simulink model "modelo2"  (R2016a)
settings: Solver=VariableStepAuto  StartTime=0.0  StopTime=2000  RelTol=1e-3
libraries: simulink x2
settings Model: Creator=Brunno  LastModifiedBy=Brunno

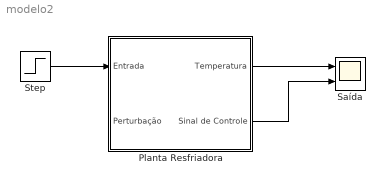
== system modelo2 ==
  Planta Resfriadora : Subsystem
  Saída : Scope  NumInputPorts=2
  Step : Step  Time=10  SampleTime=0
  wires:
  Step/1 -> Planta Resfriadora/1(Entrada)
  Planta Resfriadora/1(Temperatura) -> Saída/1
  Planta Resfriadora/2(Sinal de Controle) -> Saída/2

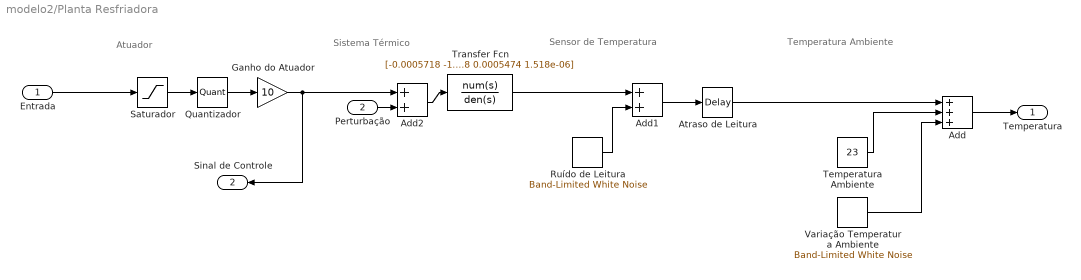
== system modelo2/Planta Resfriadora ==
  note: Temperatura Ambiente
  note: Sistema Térmico
  note: Atuador
  note: Sensor de Temperatura
  Entrada : Inport
  Perturbação : Inport  Port=2
  Add : Sum  Inputs=+++
  Add1 : Sum
  Add2 : Sum
  Atraso de Leitura : TransportDelay
  Ganho do Atuador : Gain  Gain=10
  Quantizador : Quantizer  QuantizationInterval=1/255
  Ruído de Leitura : simulink/Sources/Band-Limited White Noise  Cov=[0.001]  Ts=20  seed=[23341]
  Saturador : Saturate  UpperLimit=1  LowerLimit=0
  Temperatura Ambiente : Constant  Value=23
  Transfer Fcn : TransferFcn  Numerator=[-0.0005718 -1.226e-06]  Denominator=[1 0.04098 0.0005474 1.518e-06]
  Variação Temperatura Ambiente : simulink/Sources/Band-Limited White Noise  Cov=[1]  Ts=1000  seed=[23341]
  Temperatura : Outport
  Sinal de Controle : Outport  Port=2
  wires:
  Temperatura Ambiente/1 -> Add/2
  Entrada/1 -> Saturador/1
  Saturador/1 -> Quantizador/1
  Quantizador/1 -> Ganho do Atuador/1
  Variação Temperatura Ambiente/1 -> Add/3
  Atraso de Leitura/1 -> Add/1
  Add/1 -> Temperatura/1
  Add1/1 -> Atraso de Leitura/1
  Ruído de Leitura/1 -> Add1/2
  Transfer Fcn/1 -> Add1/1
  Add2/1 -> Transfer Fcn/1
  Ganho do Atuador/1 -> Add2/1, Sinal de Controle/1
  Perturbação/1 -> Add2/2
